simulink model "iir"  (R2016a)
settings: Solver=FixedStepDiscrete  SolverMode=SingleTasking  StartTime=0.0  StopTime=0.05  RelTol=1e-3
libraries: dsparch4 x2, dspsrcs4 x2
Description:
  | The purpuse of this model is to compare the performances of two fixed-point IIR filters; one is well designed and the another is bad designed to avoid overflow problems.
settings Model: Creator=Rodrigo Gonzalez  LastModifiedBy=rodralez
settings SolverCC: AutoInsertRateTranBlk=on
settings DataIOCC: LimitDataPoints=on  SaveOutput=off  SignalLogging=off  SaveTime=off
settings DebuggingCC: AlgebraicLoopMsg=error  SingleTaskRateTransMsg=error  AllowSymbolicDim=off
settings ConfigComp: CovModelRefEnable=Off  CovSFcnEnable=off

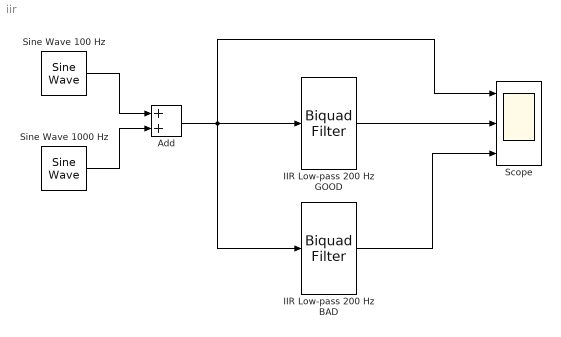
== system iir ==
  Add : Sum
  IIR Low-pass 200 Hz BAD : dsparch4/Biquad Filter  IIRFiltStruct=Direct form II  CoeffSource=Specify via dialog  BiQuadCoeffs=Hd.sosMatrix  a0Flag=Warning  IC=0  ICnum=0  ICden=0  denAccumFracLength=30  prodOutputMode=Binary point scaling  prodOutputWordLength=16  prodOutputFracLength=16  denProdOutputFracLength=16  secondMemoryFracLength=15  roundingMode=Floor  overflowMode=off  ScaleValues=Hd.ScaleValues  optimizeScaleValues=on  ScaleValueMode=Specify via input port (g)  scaleValueFracLength=14  stageInputMode=Binary point scaling  stageInputWordLength=16  stageInputFracLength=15  FilterSource=Specify via dialog  FilterObject=BQF
      settings: LockScale=on
  IIR Low-pass 200 Hz GOOD : dsparch4/Biquad Filter  IIRFiltStruct=Direct form II  CoeffSource=Specify via dialog  BiQuadCoeffs=Hd.sosMatrix  a0Flag=Warning  IC=0  ICnum=0  ICden=0  accumMode=Slope and bias scaling  accumWordLength=40  accumFracLength=32  denAccumFracLength=32  prodOutputMode=Slope and bias scaling  prodOutputWordLength=32  prodOutputFracLength=30  denProdOutputFracLength=30  secondMemoryFracLength=15  roundingMode=Round  overflowMode=on  ScaleValues=Hd.ScaleValues  optimizeScaleValues=on  ScaleValueMode=Specify via input port (g)  scaleValueFracLength=14  stageInputMode=Binary point scaling  stageInputWordLength=16  stageInputFracLength=15  FilterSource=Specify via dialog  FilterObject=BQF
      settings: LockScale=on
  Scope : Scope  NumInputPorts=3
  Sine Wave 100 Hz : dspsrcs4/Sine Wave  Amplitude=1  Frequency=100  Phase=0  SampleMode=Discrete  OutComplex=Real  CompMethod=Table lookup  TableSize=Speed  SampleTime=1/50000  SamplesPerFrame=1  ResetState=Restart at time zero  OutputFrames=off  dataType=Fixed-point  wordLen=12  udDataType=sfix(16)  fracBitsMode=Best precision  numFracBits=11  OutDataTypeStr=fixdt(1,12)  LastOutDataTypeStr=fixdt(1,12)
  Sine Wave 1000 Hz : dspsrcs4/Sine Wave  Amplitude=1  Frequency=1000  Phase=0  SampleMode=Discrete  OutComplex=Real  CompMethod=Table lookup  TableSize=Speed  SampleTime=1/50000  SamplesPerFrame=1  ResetState=Restart at time zero  OutputFrames=off  dataType=Fixed-point  wordLen=12  udDataType=sfix(16)  fracBitsMode=Best precision  numFracBits=10  OutDataTypeStr=fixdt(1,12)  LastOutDataTypeStr=fixdt(1,12)
  wires:
  Sine Wave 100 Hz/1 -> Add/1
  Sine Wave 1000 Hz/1 -> Add/2
  IIR Low-pass 200 Hz GOOD/1 -> Scope/2
  Add/1 -> IIR Low-pass 200 Hz BAD/1, IIR Low-pass 200 Hz GOOD/1, Scope/1
  IIR Low-pass 200 Hz BAD/1 -> Scope/3
